simulink model "rlhighDynamicAcc"  (R2022b)
settings: Solver=ode4  StartTime=0.0  StopTime=inf  FixedStep=fixed_step_size  RelTol=1e-3  EnableMultiTasking=on
PreLoadFcn:
  | filepath  = fileparts(get_param(bdroot, 'FileName'))
  | cd(filepath);
InitFcn:
  | [filepath,name,ext] = fileparts(get_param(bdroot, 'FileName'));
  | InitFileName=[name,'_init.m'];
  | cd(filepath);
  | open_system(name);
  | % 命令旋钮
  | constant_block_path =[name '/cmd4UAVs'];
  | set_param(constant_block_path,'Value','0');
  | % 滑杆位置
  | constant_block_path = [name '/x_d'];
  | set_param(constant_block_path,'Value','0');
  | constant_block_path = [name '/y_d'];
  | set_param(constant_block_path,'Value','0');
  | constant_block_path = [name '/z_d'];
  | set_param(constant_block_path,'Value','-1.0');
  | constant_block_path = [name '/yaw_d'];
  | set_param(constant_block_path,'Value','0');
  | save_system(name);
  | try
  | run(InitFileName);
  | end
values from neighbouring files (symbols this model uses):
  MAX_ACC_HOR = 4.0    (= 4)    [rlhighDynamicAcc_init.m]
  MAX_POS_ERR = 4.0    (= 4)    [rlhighDynamicAcc_init.m]
  MAX_YAW_RATE = 1.0    (= 1)    [rlhighDynamicAcc_init.m]
  Pos_Y_I = 0.0    (= 0)    [rlhighDynamicAcc_init.m]
  Pos_Y_P = 1.0    (= 1)    [rlhighDynamicAcc_init.m]
  Pos_Z_P = 1.0    (= 1)    [rlhighDynamicAcc_init.m]
  Saturation_I_ah = 1.0    (= 1)    [rlhighDynamicAcc_init.m]
  Ts = fixed_step_size    (= 0.02)    [rlhighDynamicAcc_init.m]
  Vel_Y_I = 0.5    [rlhighDynamicAcc_init.m]
  Vel_Y_P = 2.0    (= 2)    [rlhighDynamicAcc_init.m]
  Yaw_I = 0.1    [rlhighDynamicAcc_init.m]
  Yaw_P = 1.0    (= 1)    [rlhighDynamicAcc_init.m]
undefined symbols (not defined in the file or in its folder): DiscIntNeverNeededParam
libraries: simulink x3, pixhawk_slib_swarm x3, rllib x1
settings Model: Creator=dream  LastModifiedBy=admin
settings SolverCC: AlgebraicLoopSolver=TrustRegion
settings DataIOCC: SaveFormat=Array  ReturnWorkspaceOutputs=off
settings OptimizationCC: BlockReduction=off  BooleanDataType=off  ZeroExternalMemoryAtStartup=off  ZeroInternalMemoryAtStartup=off
settings DebuggingCC: SaveWithParameterizedLinksMsg=none  UnderspecifiedInitializationDetection=Classic  MergeDetectMultiDrivingBlocksExec=none  SignalResolutionControl=TryResolveAllWithWarning  MultiTaskDSMMsg=warning  MultiTaskCondExecSysMsg=none  UnconnectedInputMsg=warning  UnconnectedOutputMsg=warning  UnconnectedLineMsg=warning  SFMachineParentedDataDiag=warning  ArithmeticOperatorsInVariantConditions=warning
settings HardwareCC: TargetBitPerPointer=64  TargetBitPerSizeT=64  TargetBitPerPtrDiffT=64  TargetLongLongMode=on  TargetIntDivRoundTo=Zero  TargetEndianess=LittleEndian  TargetWordSize=64  TargetHWDeviceType=MATLAB Host  ProdEqTarget=off
settings ModelReferenceCC: EnableRefExpFcnMdlSchedulingChecks=on  PropagateSignalLabelsOutOfModel=off
settings SFSimCC: SimUseLocalCustomCode=off  CustomCodeUndefinedFunction=UseInterfaceOnly  SimTargetLang=C++
settings RTWCC: PackageGeneratedCodeAndArtifacts=on  PackageName=RflyUdpExe  RTWUseLocalCustomCode=off  CustomLibrary=quat_mt.lib vrpn_mt.lib  BuildConfiguration=Faster Runs  TargetLang=C++
settings GRTTargetCC: TargetLangStandard=C++03 (ISO)  CodeInterfacePackaging=C++ class  MultiInstanceErrorCode=None

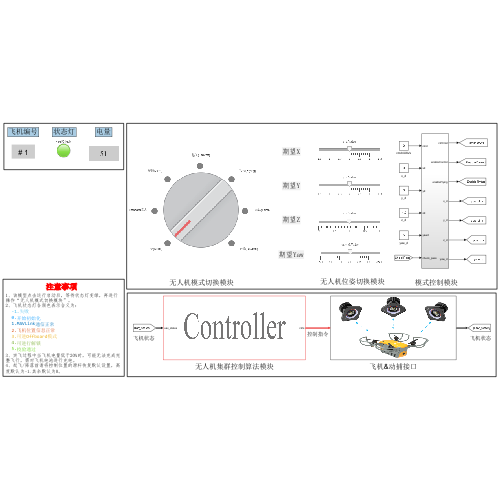
[thumbnail: Simulink's stored preview of the top-level diagram]
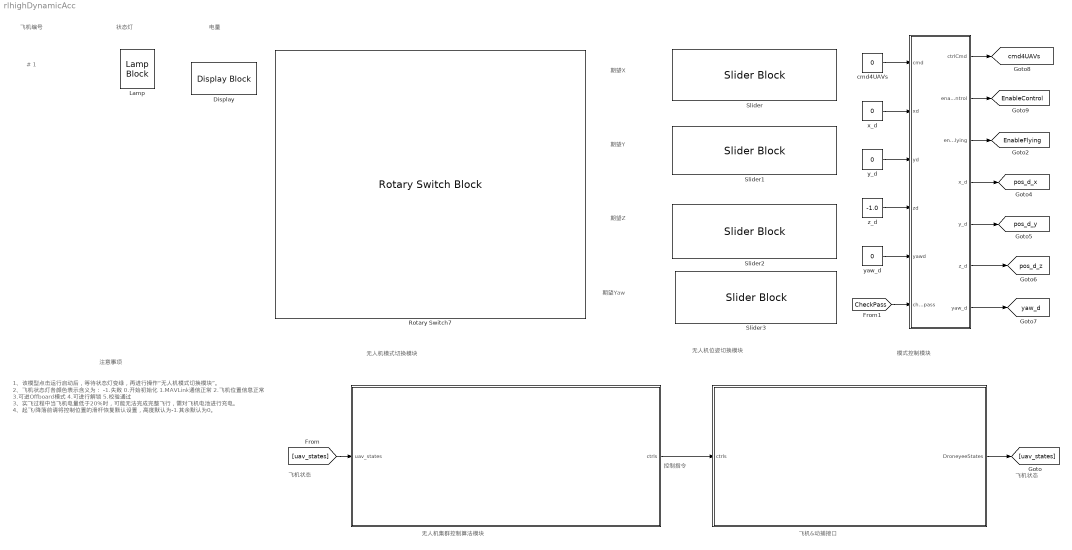
== system rlhighDynamicAcc ==
  note: 1、该模型点击运行启动后，等待状态灯变绿，再进行操作“无人机模式切换模块”。
      | 2、飞机状态灯各颜色表示含义为：
      | -1.失败
      | 0.开始初始化
      | 1.MAVLink通信正常
      | 2.飞机位置信息正常
      | 3.可进Offboard模式
      | 4.可进行解锁
      | 5.校验通过
      | 3、实飞过程中当飞机电量低于20%时，可能无法完成完整飞行，需对飞机电池进行充电。
      | 4、起飞/降落前请将控制位置的滑杆恢复默认设置，高度默认为-1.其余默认为0。
  note: 注意事项
  note: 控制指令
  note: 飞机&动捕接口
  note: 飞机编号
  note: 状态灯
  note: 电量
  note: # 1
  note: 无人机集群控制算法模块
  note: 飞机状态
  note: 模式控制模块
  note: 无人机模式切换模块
  note: 飞机状态
  note: 无人机位姿切换模块
  note: 期望Y
  note: 期望Z
  note: 期望X
  note: 期望Yaw
  " " : Subsystem
      mask Display: image('Controller.png');
  "   " : Subsystem
      mask Display: image('Odc_Sys.png');
  "    " : Subsystem
  Display : DisplayBlock  LabelPosition=Hide  Format=long
  Lamp : LampBlock
  Rotary Switch7 : RotarySwitchBlock  LabelPosition=Hide
      settings: Values={{'无(None)', 'Offboard模式', '解锁(Arm)', '起飞(Takeoff)', '飞行(Flying)', '着陆(Land)', '上锁(Disarm)'}, [0 8 4 256 512 1024 128]}
  Slider : SliderBlock  ScaleMin=-1.5  ScaleMax=1.5  TickInterval=0.5
  Slider1 : SliderBlock  ScaleMin=-1.5  ScaleMax=1.5  TickInterval=0.5
  Slider2 : SliderBlock  ScaleMin=-2  ScaleMax=0  TickInterval=0.5
  Slider3 : SliderBlock  ScaleMin=-3.1  ScaleMax=3.1  TickInterval=1
  cmd4UAVs : Constant  Value=0
  x_d : Constant  Value=0
  y_d : Constant  Value=0
  yaw_d : Constant  Value=0
  z_d : Constant  Value=-1.0
  tag scope: EnableControl=global, EnableFlying=global, cmd4UAVs=global, pos_d_x=global, pos_d_y=global, pos_d_z=global, yaw_d=global
  wires:
  " "/1(ctrls) -> "   "/1(ctrls)
  "   "/1(DroneyeeStates) -> [uav_states]
  [uav_states] -> " "/1(uav_states)
  "    "/6(z_d) -> [pos_d_z]
  "    "/3(enableFlying) -> [EnableFlying]
  "    "/2(enableControl) -> [EnableControl]
  "    "/1(ctrlCmd) -> [cmd4UAVs]
  [CheckPass] -> "    "/6(check_pass)
  "    "/4(x_d) -> [pos_d_x]
  z_d/1 -> "    "/4(zd)
  yaw_d/1 -> "    "/5(yawd)
  cmd4UAVs/1 -> "    "/1(cmd)
  y_d/1 -> "    "/3(yd)
  "    "/7(yaw_d) -> [yaw_d]
  "    "/5(y_d) -> [pos_d_y]
  x_d/1 -> "    "/2(xd)

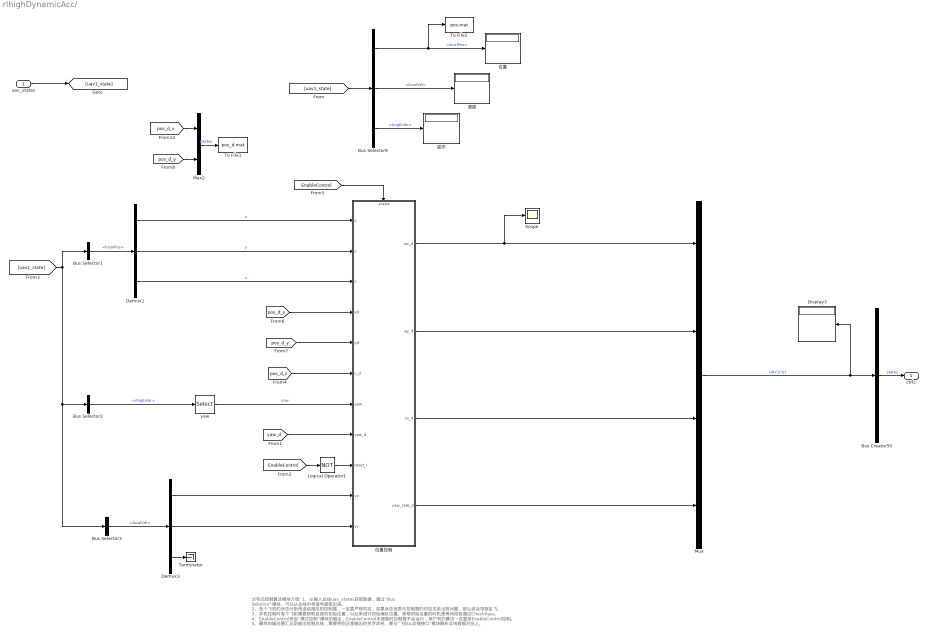
== system rlhighDynamicAcc/  ==
  note: 分布式控制算法模块介绍:
      |
      | 1、从输入总线uav_states获取数据，通过“Bus Selector”模块，可以从总线中将信号提取出来。
      | 2、各个飞机的状态分别传送给相应的控制器，一定要严格对应，如果状态信息与控制器的对应关系出现问题，那么就会导致乱飞。
      | 3、多机控制时每个飞机需要获取自身的初始位置，以此来进行初始编队位置。获取初始位置的时机是等待校验通过CheckPass。
      | 4、EnableControl来自“模式控制”模块的输出，EnableControl未使能时控制器不会运行，用户写的算法一定要受EnableControl控制。
      | 5、最终的输出要汇总到输出控制总线，需要特别注意输出的名字命名，要与“飞机&动捕接口”模块解析总线数据对应上。
  uav_states : Inport
  Bus Creator50 : BusCreator  Inputs=1
  Bus Selector1 : BusSelector  OutputSignals=localPos
  Bus Selector2 : BusSelector  OutputSignals=AngEular
  Bus Selector3 : BusSelector  OutputSignals=localVel
  Bus Selector9 : BusSelector  OutputSignals=localPos,localVel,AngEular
  Demux1 : Demux  Outputs=3
  Demux3 : Demux  Outputs=3
  Display3 : Display
  Logical Operator1 : Logic  Operator=NOT  AllPortsSameDT=off  OutDataTypeStr=boolean
  Mux : Mux
  Mux2 : Mux  Inputs=2
  Scope : Scope
  Terminator : Terminator
  To File1 : ToFile  Filename=pos_d.mat  SaveFormat=Timeseries
  To File2 : ToFile  Filename=pos.mat  SaveFormat=Timeseries
  yaw : Selector  InputPortWidth=3  IndexOptions=Index vector (dialog)  Indices=[3]  OutputSizes=1
  位置 : Display
  位置控制 : Subsystem
  姿态 : Display
  速度 : Display
  ctrls : Outport  VectorParamsAs1DForOutWhenUnconnected=off
  wires:
  Bus Creator50/1 -> ctrls/1  "states"
  Mux/1 -> Display3/1, Bus Creator50/1  "UAV1Ctrl"
  [uav1_state] -> Bus Selector1/1, Bus Selector3/1, Bus Selector2/1
  Demux1/1 -> 位置控制/1(x)  "x"
  Demux1/2 -> 位置控制/2(y)  "y"
  Demux1/3 -> 位置控制/3(z)  "z"
  Bus Selector1/1 -> Demux1/1  "<localPos>"
  yaw/1 -> 位置控制/7(yaw)  "yaw"
  Bus Selector2/1 -> yaw/1  "<AngEular>"
  位置控制/3(vz_d) -> Mux/3
  位置控制/4(yaw_rate_d) -> Mux/4
  Bus Selector9/3 -> 姿态/1  "<AngEular>"
  Bus Selector9/2 -> 速度/1  "<localVel>"
  Bus Selector9/1 -> To File2/1, 位置/1  "<localPos>"
  [uav1_state] -> Bus Selector9/1
  uav_states/1 -> [uav1_state]
  [EnableControl] -> 位置控制/Enable
  [yaw_d] -> 位置控制/8(yaw_d)
  [pos_d_z] -> 位置控制/6(z_d)
  [pos_d_y] -> 位置控制/5(yd)
  [pos_d_x] -> 位置控制/4(xd)
  Logical Operator1/1 -> 位置控制/9(reset_i)
  [EnableControl] -> Logical Operator1/1
  Demux3/3 -> Terminator/1
  Bus Selector3/1 -> Demux3/1  "<localVel>"
  Demux3/1 -> 位置控制/10(vx)
  Demux3/2 -> 位置控制/11(vy)
  位置控制/1(ax_d) -> Mux/1, Scope/1
  位置控制/2(ay_d) -> Mux/2
  [pos_d_x] -> Mux2/1
  [pos_d_y] -> Mux2/2
  Mux2/1 -> To File1/1  "states"

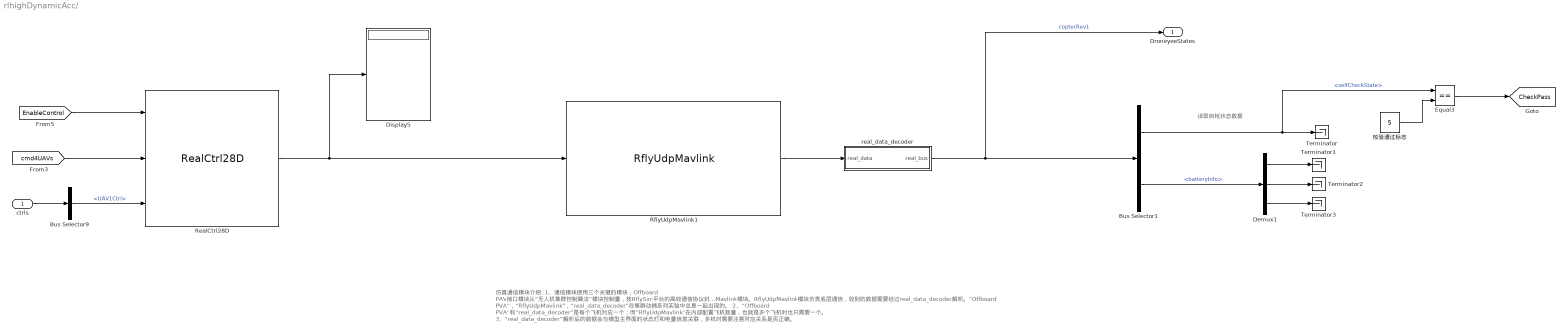
== system rlhighDynamicAcc/    ==
  note: 读取自检状态数据
  note: 仿真通信模块介绍:
      |
      | 1、通信模块使用三个关键的模块，Offboard PAV接口模块从“无人机集群控制算法”模块控制量，按RflySim平台的高效通信协议封装后传递给RflyUdpMavlink模块。RflyUdpMavlink模块负责底层通信，收到的数据需要经过real_data_decoder解析。“Offboard PVA”，“RflyUdpMavlink”，“real_data_decoder”在集群动捕系列实验中总是一起出现的。
      | 2、“Offboard PVA”和“real_data_decoder”是每个飞机对应一个；而“RflyUdpMavlink”在内部配置飞机数量，也就是多个飞机时也只需要一个。
      | 3、“real_data_decoder”解析后的数据会与模型主界面的状态灯和电量信息关联，多机时需要注意对应关系是否正确。
  ctrls : Inport
  Bus Selector1 : BusSelector  OutputSignals=selfCheckState,batteryInfo
  Bus Selector9 : BusSelector  OutputSignals=UAV1Ctrl
  Demux1 : Demux  Outputs=3
  Display5 : Display
  Equal3 : RelationalOperator  Operator===  OutDataTypeStr=boolean  RndMeth=Simplest  InputSameDT=off
  RealCtrl28D : pixhawk_slib_swarm/RealCtrl28D  isX=off  isY=off  isZ=off  isVx=off  isVy=off  isVz=on  isAx=on  isAy=on  isAz=off  isYaw=off  isYawRate=on  EnIdxList=[1]  isRcc=off  isForce=off  SamTime=-1
      settings: SourceProductName=Pixhawk Target Blocks
  RflyUdpMavlink1 : pixhawk_slib_swarm/RflyUdpMavlink  idx=1  ip1=127.0.0.1  ip=192.168.151.103  num=1  port=15501  Gps=[40.1540302,116.2593683,50.0]  udpmode=Mavlink_Real  T=1/50  isSame=off
      settings: SourceProductName=Pixhawk Target Blocks
  Terminator{,1..3} (4 alike) : Terminator
  real_data_decoder : Subsystem
      mask DialogControl Control2 Prompt: (Add text here)
  校验通过标志 : Constant  Value=5
  DroneyeeStates : Outport  VectorParamsAs1DForOutWhenUnconnected=off
  tag scope: CheckPass=global
  wires:
  RealCtrl28D/1 -> RflyUdpMavlink1/1, Display5/1
  RflyUdpMavlink1/1 -> real_data_decoder/1(real_data)
  real_data_decoder/1(real_bus) -> DroneyeeStates/1, Bus Selector1/1  "copterRev1"
  Bus Selector1/1 -> Equal3/1, Terminator/1  "<selfCheckState>"
  Demux1/3 -> Terminator3/1
  Demux1/2 -> Terminator2/1
  Demux1/1 -> Terminator1/1
  Bus Selector1/2 -> Demux1/1  "<batteryInfo>"
  Bus Selector9/1 -> RealCtrl28D/3  "<UAV1Ctrl>"
  [EnableControl] -> RealCtrl28D/1
  [cmd4UAVs] -> RealCtrl28D/2
  ctrls/1 -> Bus Selector9/1
  校验通过标志/1 -> Equal3/2
  Equal3/1 -> [CheckPass]

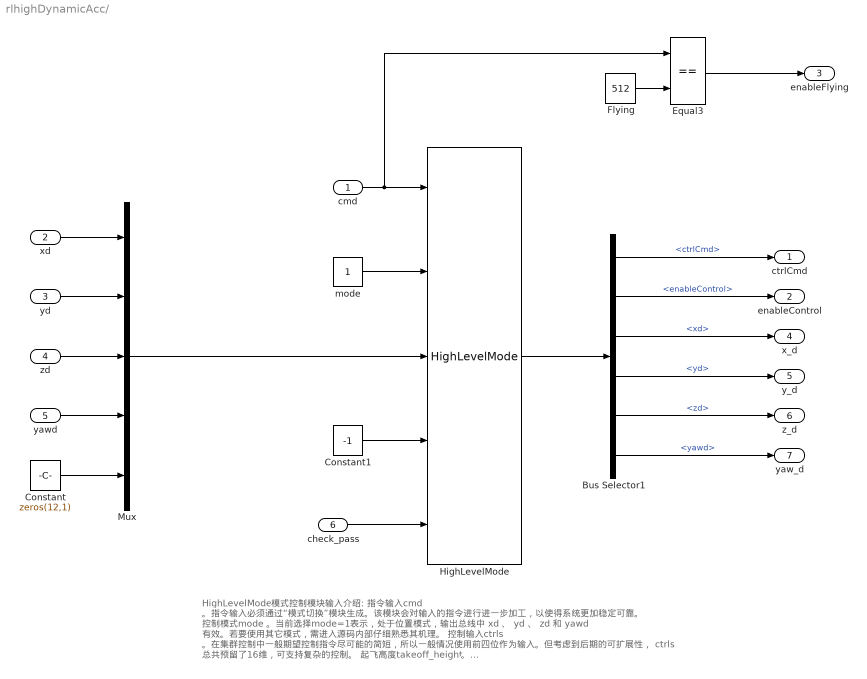
== system rlhighDynamicAcc/     ==
  note: HighLevelMode模式控制模块输入介绍:
      | 指令输入cmd 。指令输入必须通过“模式切换”模块生成。该模块会对输入的指令进行进一步加工，以使得系统更加稳定可靠。
      | 控制模式mode 。当前选择mode=1表示，处于位置模式，输出总线中 xd 、 yd 、 zd 和 yawd 有效。若要使用其它模式，需进入源码内部仔细熟悉其机理。
      | 控制输入ctrls 。在集群控制中一般期望控制指令尽可能的简短，所以一般情况使用前四位作为输入。但考虑到后期的可扩展性， ctrls 总共预留了16维，可支持复杂的控制。
      | 起飞高度takeoff_height。 起飞高度是指当用户将“模式切换”模块旋转到起飞时，飞机将自动起飞到的高度。该高度以向下为正，与无人机的 NED 坐标系兼容。在室内场景下，建议默认高度为1m，即在 MATLAB 中设置数值为-1。
      | 飞机状态校验是否通过check_pass 。 所有飞机校验通过才算通过，该信号来自飞机&动捕接口。
      | HighLevelMode模式控制模块输出介绍:
      | “模式控制”模块的输出是一个总线，MATLAB在从总线中提取数据时会显示总线中有哪些类型的数据，这样可以便于用户选择所需要的数据。
  cmd : Inport
  xd : Inport  Port=2
  yd : Inport  Port=3
  zd : Inport  Port=4
  yawd : Inport  Port=5
  check_pass : Inport  Port=6
  Bus Selector1 : BusSelector  OutputSignals=ctrlCmd,enableControl,xd,yd,zd,yawd
  Constant : Constant  Value=zeros(12,1)
  Constant1 : Constant  Value=-1
  Equal3 : RelationalOperator  Operator===  OutDataTypeStr=boolean  RndMeth=Simplest  InputSameDT=off
  Flying : Constant  Value=512
  HighLevelMode : pixhawk_slib_swarm/HighLevelMode
      settings: SourceProductName=Pixhawk Target Blocks
  Mux : Mux  Inputs=5
  mode : Constant
  ctrlCmd : Outport  VectorParamsAs1DForOutWhenUnconnected=off
  enableControl : Outport  Port=2  VectorParamsAs1DForOutWhenUnconnected=off
  enableFlying : Outport  Port=3  VectorParamsAs1DForOutWhenUnconnected=off
  x_d : Outport  Port=4  VectorParamsAs1DForOutWhenUnconnected=off
  y_d : Outport  Port=5  VectorParamsAs1DForOutWhenUnconnected=off
  z_d : Outport  Port=6  VectorParamsAs1DForOutWhenUnconnected=off
  yaw_d : Outport  Port=7  VectorParamsAs1DForOutWhenUnconnected=off
  wires:
  Mux/1 -> HighLevelMode/3
  Bus Selector1/5 -> z_d/1  "<zd>"
  Bus Selector1/3 -> x_d/1  "<xd>"
  Bus Selector1/2 -> enableControl/1  "<enableControl>"
  Constant1/1 -> HighLevelMode/4
  Bus Selector1/1 -> ctrlCmd/1  "<ctrlCmd>"
  yawd/1 -> Mux/4
  HighLevelMode/1 -> Bus Selector1/1
  Constant/1 -> Mux/5
  check_pass/1 -> HighLevelMode/5
  xd/1 -> Mux/1
  zd/1 -> Mux/3
  Bus Selector1/4 -> y_d/1  "<yd>"
  mode/1 -> HighLevelMode/2
  yd/1 -> Mux/2
  Bus Selector1/6 -> yaw_d/1  "<yawd>"
  Equal3/1 -> enableFlying/1
  Flying/1 -> Equal3/2
  cmd/1 -> Equal3/1, HighLevelMode/1

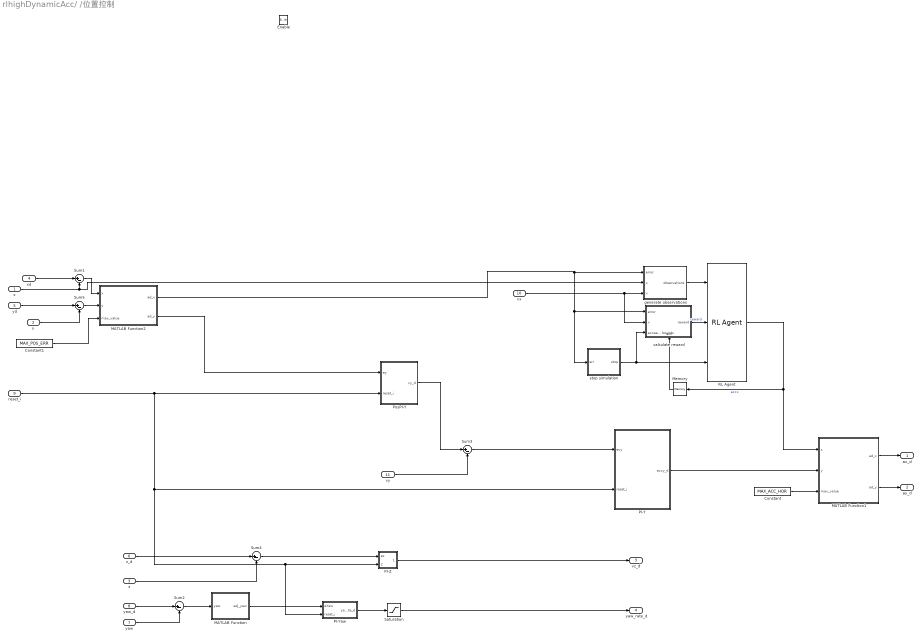
== system rlhighDynamicAcc/ /位置控制 ==
  x : Inport
  y : Inport  Port=2
  z : Inport  Port=3
  xd : Inport  Port=4
  yd : Inport  Port=5
  z_d : Inport  Port=6
  yaw : Inport  Port=7
  yaw_d : Inport  Port=8
  reset_i : Inport  Port=9
  vx : Inport  Port=10
  vy : Inport  Port=11
  Enable : EnablePort
  Constant : Constant  Value=MAX_ACC_HOR
  Constant1 : Constant  Value=MAX_POS_ERR
  MATLAB Function : MATLAB Function  TreatAsAtomicUnit=on
  MATLAB Function1 : MATLAB Function  TreatAsAtomicUnit=on
  MATLAB Function2 : MATLAB Function  TreatAsAtomicUnit=on
  Memory : Memory
  PI-Y : Subsystem
  PI-Yaw : Subsystem
  PI-Z : Subsystem
  PosPI-Y : Subsystem
  RL Agent : rllib/RL Agent  Agent=agent  ExternalActionAsInput=off  ProvideLastAction=off  ProvideCumRwd=off  TreatAsDirectFeedthrough=on  UseStrictObservationDataTypes=off
  Saturation : Saturate  UpperLimit=MAX_YAW_RATE  LowerLimit=-MAX_YAW_RATE
  Sum{1..5} (5 alike) : Sum  Inputs=|+-
  calculate reward : Subsystem
      settings: PortSchema="{\"entries\":[{\"content\":{\"sides\":[{\"content\":{\"connectorIds\":[\"In1\",\"In2\",\"In3\"]},\"type\":\"ConnectorPlacement.EquallySpacedRectSide\",\"uuid\":\"a6831b4c-c5e4-4b81-8e40-7fc4b7dad633\"},{\"content\":{\"connectorIds\":[\"Out1\"],\"side\":\"RIGHT\"},\"type\":\"ConnectorPlacement.EquallySpacedRectSide\",\"uuid\":\"8e922aec-ef45-4070-9445-bf1f36bf8a17\"},{\"content\":{\"connectorIds\":[],\"side\":\"TOP\"},\"type\":\"ConnectorPlacement.EquallySpacedRectSide\",\"uuid\":\"70fa4f95-2353-478a-a00d-3d58ec9167ce\"},{\"content\":{\"connectorIds\":[\"In4\"],\"side\":\"BOTTOM\"},\"type\":\"ConnectorPlacement.EquallySpacedRectSide\",\"uuid\":\"92073c7e-e113-4538-8fec-17539d6aadbe\"}]},\"type\":\"ConnectorPlacement.EquallySpacedConnector\",\"uuid\":\"a5a5b4e0-4f16-4179-a493-15187e3b2ccc\"}],\"packageUris\":[\"http://schema.mathworks.com/mf0/Connector/R2020b\"],\"version\":\"1.0\"}"
  generate observations : Subsystem
  stop simulation : Subsystem
  ax_d : Outport  VectorParamsAs1DForOutWhenUnconnected=off
  ay_d : Outport  Port=2  VectorParamsAs1DForOutWhenUnconnected=off
  vz_d : Outport  Port=3  VectorParamsAs1DForOutWhenUnconnected=off
  yaw_rate_d : Outport  Port=4  VectorParamsAs1DForOutWhenUnconnected=off
  wires:
  yaw_d/1 -> Sum2/1
  MATLAB Function/1(adj_yaw) -> PI-Yaw/1(eYaw)
  PI-Yaw/1(yawRate_d) -> Saturation/1
  z_d/1 -> Sum4/1
  PI-Z/1(vy_d) -> vz_d/1
  Saturation/1 -> yaw_rate_d/1
  z/1 -> Sum4/2
  yaw/1 -> Sum2/2
  Sum4/1 -> PI-Z/1(ez)
  Sum2/1 -> MATLAB Function/1(yaw)
  MATLAB Function1/1(ad_x) -> ax_d/1
  MATLAB Function1/2(ad_y) -> ay_d/1
  vy/1 -> Sum3/2
  Sum3/1 -> PI-Y/1(evy)
  PosPI-Y/1(vy_d) -> Sum3/1
  PI-Y/1(accy_d) -> MATLAB Function1/2(y)
  Constant/1 -> MATLAB Function1/3(max_value)
  Constant1/1 -> MATLAB Function2/3(max_value)
  xd/1 -> Sum1/1
  yd/1 -> Sum5/1
  Sum5/1 -> MATLAB Function2/2(y)
  Sum1/1 -> MATLAB Function2/1(x)
  MATLAB Function2/2(ad_y) -> PosPI-Y/1(ey)
  x/1 -> generate observations/2(x), Sum1/2
  reset_i/1 -> PI-Z/2(reset_i), PI-Yaw/2(reset_i), PI-Y/2(reset_i), PosPI-Y/2(reset_i)
  y/1 -> Sum5/2
  vx/1 -> calculate reward/2(v), generate observations/3(v)
  MATLAB Function2/1(ad_x) -> generate observations/1(error), calculate reward/1(error), stop simulation/1(err)
  generate observations/1(observations) -> RL Agent/1
  stop simulation/1(stop) -> calculate reward/3(exceeds bounds), RL Agent/3
  RL Agent/1 -> MATLAB Function1/1(x), Memory/1  "accx"
  calculate reward/1(reward) -> RL Agent/2  "reward"
  Memory/1 -> calculate reward/4(acc)

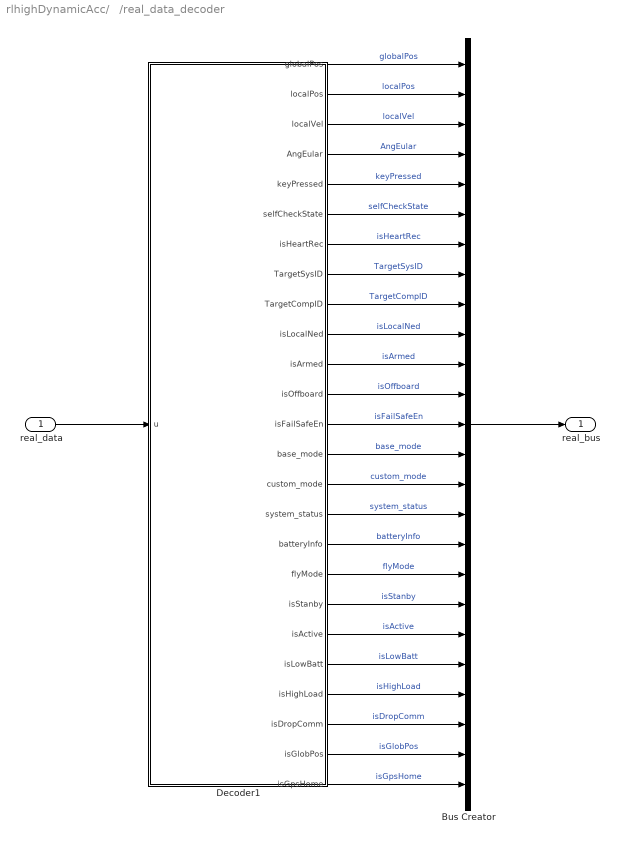
== system rlhighDynamicAcc/   /real_data_decoder ==
  real_data : Inport
  Bus Creator : BusCreator  Inputs=25
  Decoder1 : MATLAB Function  TreatAsAtomicUnit=on
  real_bus : Outport  VectorParamsAs1DForOutWhenUnconnected=off
  wires:
  Decoder1/3(localVel) -> Bus Creator/3  "localVel"
  Decoder1/15(custom_mode) -> Bus Creator/15  "custom_mode"
  Decoder1/21(isLowBatt) -> Bus Creator/21  "isLowBatt"
  Decoder1/9(TargetCompID) -> Bus Creator/9  "TargetCompID"
  Decoder1/18(flyMode) -> Bus Creator/18  "flyMode"
  Decoder1/16(system_status) -> Bus Creator/16  "system_status"
  Decoder1/5(keyPressed) -> Bus Creator/5  "keyPressed"
  real_data/1 -> Decoder1/1(u)
  Bus Creator/1 -> real_bus/1
  Decoder1/14(base_mode) -> Bus Creator/14  "base_mode"
  Decoder1/22(isHighLoad) -> Bus Creator/22  "isHighLoad"
  Decoder1/25(isGpsHome) -> Bus Creator/25  "isGpsHome"
  Decoder1/24(isGlobPos) -> Bus Creator/24  "isGlobPos"
  Decoder1/19(isStanby) -> Bus Creator/19  "isStanby"
  Decoder1/20(isActive) -> Bus Creator/20  "isActive"
  Decoder1/12(isOffboard) -> Bus Creator/12  "isOffboard"
  Decoder1/10(isLocalNed) -> Bus Creator/10  "isLocalNed"
  Decoder1/8(TargetSysID) -> Bus Creator/8  "TargetSysID"
  Decoder1/13(isFailSafeEn) -> Bus Creator/13  "isFailSafeEn"
  Decoder1/4(AngEular) -> Bus Creator/4  "AngEular"
  Decoder1/11(isArmed) -> Bus Creator/11  "isArmed"
  Decoder1/23(isDropComm) -> Bus Creator/23  "isDropComm"
  Decoder1/7(isHeartRec) -> Bus Creator/7  "isHeartRec"
  Decoder1/17(batteryInfo) -> Bus Creator/17  "batteryInfo"
  Decoder1/6(selfCheckState) -> Bus Creator/6  "selfCheckState"
  Decoder1/1(globalPos) -> Bus Creator/1  "globalPos"
  Decoder1/2(localPos) -> Bus Creator/2  "localPos"

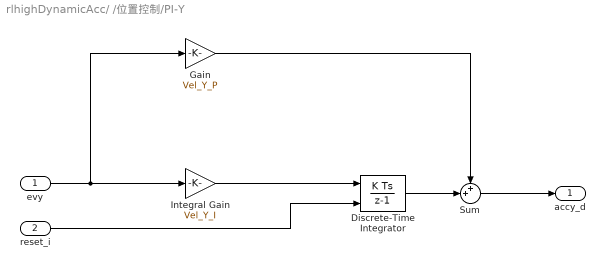
== system rlhighDynamicAcc/ /位置控制/PI-Y ==
  evy : Inport
  reset_i : Inport  Port=2
  Discrete-Time Integrator : DiscreteIntegrator  ExternalReset=level  SampleTime=-1  LimitOutput=on  UpperSaturationLimit=Saturation_I_ah  LowerSaturationLimit=-Saturation_I_ah  ICPrevOutput=DiscIntNeverNeededParam  ICPrevScaledInput=DiscIntNeverNeededParam
  Gain : Gain  Gain=Vel_Y_P
  Integral Gain : Gain  DisableCoverage=on  Gain=Vel_Y_I
  Sum : Sum  Inputs=++|
  accy_d : Outport  InitialOutput=0  VectorParamsAs1DForOutWhenUnconnected=off
  wires:
  evy/1 -> Gain/1, Integral Gain/1
  Integral Gain/1 -> Discrete-Time Integrator/1
  Gain/1 -> Sum/1
  Sum/1 -> accy_d/1
  Discrete-Time Integrator/1 -> Sum/2
  reset_i/1 -> Discrete-Time Integrator/2

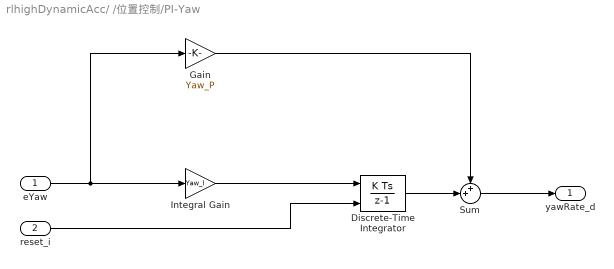
== system rlhighDynamicAcc/ /位置控制/PI-Yaw ==
  eYaw : Inport
  reset_i : Inport  Port=2
  Discrete-Time Integrator : DiscreteIntegrator  ExternalReset=level  SampleTime=-1  LimitOutput=on  UpperSaturationLimit=Saturation_I_ah  LowerSaturationLimit=-Saturation_I_ah  ICPrevOutput=DiscIntNeverNeededParam  ICPrevScaledInput=DiscIntNeverNeededParam
  Gain : Gain  Gain=Yaw_P
  Integral Gain : Gain  DisableCoverage=on  Gain=Yaw_I
  Sum : Sum  Inputs=++|
  yawRate_d : Outport  InitialOutput=0  VectorParamsAs1DForOutWhenUnconnected=off
  wires:
  eYaw/1 -> Gain/1, Integral Gain/1
  Integral Gain/1 -> Discrete-Time Integrator/1
  Gain/1 -> Sum/1
  Sum/1 -> yawRate_d/1
  Discrete-Time Integrator/1 -> Sum/2
  reset_i/1 -> Discrete-Time Integrator/2

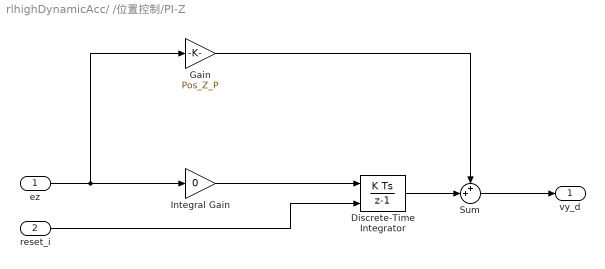
== system rlhighDynamicAcc/ /位置控制/PI-Z ==
  ez : Inport
  reset_i : Inport  Port=2
  Discrete-Time Integrator : DiscreteIntegrator  ExternalReset=level  SampleTime=-1  LimitOutput=on  UpperSaturationLimit=Saturation_I_ah  LowerSaturationLimit=-Saturation_I_ah  ICPrevOutput=DiscIntNeverNeededParam  ICPrevScaledInput=DiscIntNeverNeededParam
  Gain : Gain  Gain=Pos_Z_P
  Integral Gain : Gain  DisableCoverage=on  Gain=0
  Sum : Sum  Inputs=++|
  vy_d : Outport  InitialOutput=0  VectorParamsAs1DForOutWhenUnconnected=off
  wires:
  ez/1 -> Gain/1, Integral Gain/1
  Integral Gain/1 -> Discrete-Time Integrator/1
  Gain/1 -> Sum/1
  Sum/1 -> vy_d/1
  Discrete-Time Integrator/1 -> Sum/2
  reset_i/1 -> Discrete-Time Integrator/2

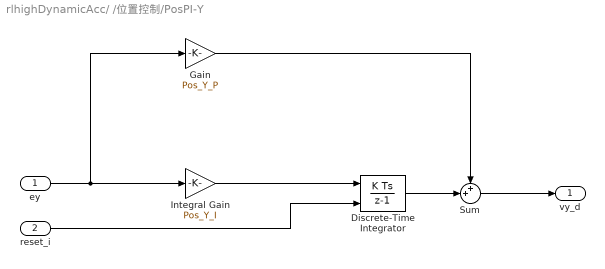
== system rlhighDynamicAcc/ /位置控制/PosPI-Y ==
  ey : Inport
  reset_i : Inport  Port=2
  Discrete-Time Integrator : DiscreteIntegrator  ExternalReset=level  SampleTime=-1  LimitOutput=on  UpperSaturationLimit=Saturation_I_ah  LowerSaturationLimit=-Saturation_I_ah  ICPrevOutput=DiscIntNeverNeededParam  ICPrevScaledInput=DiscIntNeverNeededParam
  Gain : Gain  Gain=Pos_Y_P
  Integral Gain : Gain  DisableCoverage=on  Gain=Pos_Y_I
  Sum : Sum  Inputs=++|
  vy_d : Outport  InitialOutput=0  VectorParamsAs1DForOutWhenUnconnected=off
  wires:
  ey/1 -> Gain/1, Integral Gain/1
  Integral Gain/1 -> Discrete-Time Integrator/1
  Gain/1 -> Sum/1
  Sum/1 -> vy_d/1
  Discrete-Time Integrator/1 -> Sum/2
  reset_i/1 -> Discrete-Time Integrator/2

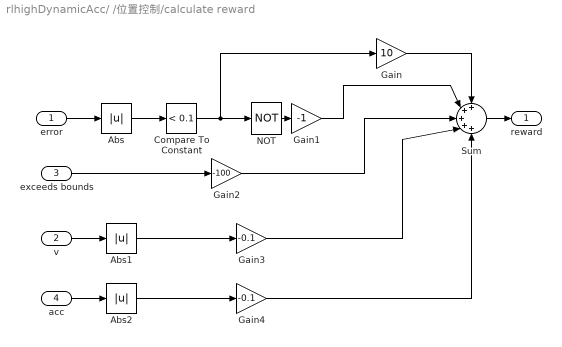
== system rlhighDynamicAcc/ /位置控制/calculate reward ==
  error : Inport
  v : Inport  Port=2
  exceeds bounds : Inport  Port=3
  acc : Inport  Port=4
  Abs : Abs  SaturateOnIntegerOverflow=off
  Abs1 : Abs  ZeroCross=off  SaturateOnIntegerOverflow=off
  Abs2 : Abs  ZeroCross=off  SaturateOnIntegerOverflow=off
  Compare To Constant : simulink/Logic and Bit Operations/Compare To Constant  relop=<  const=0.1  OutDataTypeStr=boolean
  Gain : Gain  Gain=10
  Gain1 : Gain  Gain=-1
  Gain2 : Gain  Gain=-100
  Gain3 : Gain  Gain=-0.1
  Gain4 : Gain  Gain=-0.1
  NOT : Logic  Operator=NOT  IconShape=distinctive  AllPortsSameDT=off  OutDataTypeStr=boolean
  Sum : Sum  Inputs=+++++  OutDataTypeStr=double
  reward : Outport  VectorParamsAs1DForOutWhenUnconnected=off
  wires:
  Abs/1 -> Compare To Constant/1
  Gain2/1 -> Sum/3
  Gain/1 -> Sum/1
  Compare To Constant/1 -> NOT/1, Gain/1
  Gain1/1 -> Sum/2
  Sum/1 -> reward/1
  NOT/1 -> Gain1/1
  exceeds bounds/1 -> Gain2/1
  error/1 -> Abs/1
  v/1 -> Abs1/1
  Gain3/1 -> Sum/4
  Abs1/1 -> Gain3/1
  Abs2/1 -> Gain4/1
  acc/1 -> Abs2/1
  Gain4/1 -> Sum/5

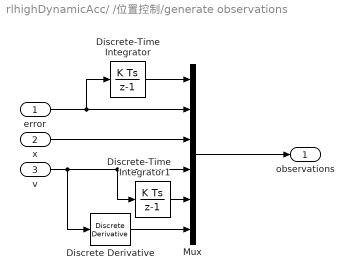
== system rlhighDynamicAcc/ /位置控制/generate observations ==
  error : Inport
  x : Inport  Port=2
  v : Inport  Port=3
  Discrete Derivative : simulink/Discrete/Discrete Derivative  gainval=0.01  ICPrevScaledInput=0.0  OutMin=[]  OutMax=[]  OutDataType=fixdt(1, 16)  OutScaling=2^-10  DoSatur=off
  Discrete-Time Integrator : DiscreteIntegrator  SampleTime=Ts  ICPrevOutput=DiscIntNeverNeededParam  ICPrevScaledInput=DiscIntNeverNeededParam
  Discrete-Time Integrator1 : DiscreteIntegrator  gainval=0.1  SampleTime=Ts  ICPrevOutput=DiscIntNeverNeededParam  ICPrevScaledInput=DiscIntNeverNeededParam
  Mux : Mux  Inputs=6
  observations : Outport  VectorParamsAs1DForOutWhenUnconnected=off
  wires:
  x/1 -> Mux/3
  Discrete-Time Integrator/1 -> Mux/1
  error/1 -> Discrete-Time Integrator/1, Mux/2
  Mux/1 -> observations/1
  v/1 -> Discrete Derivative/1, Discrete-Time Integrator1/1, Mux/4
  Discrete-Time Integrator1/1 -> Mux/5
  Discrete Derivative/1 -> Mux/6

== system rlhighDynamicAcc/ /位置控制/stop simulation ==
  err : Inport
  Abs : Abs  SaturateOnIntegerOverflow=off
  Compare To Constant : simulink/Logic and Bit Operations/Compare To Constant  relop=>  const=10  OutDataTypeStr=boolean
  stop : Outport  VectorParamsAs1DForOutWhenUnconnected=off
  wires:
  err/1 -> Abs/1
  Abs/1 -> Compare To Constant/1
  Compare To Constant/1 -> stop/1

== matlab function rlhighDynamicAcc/   /real_data_decoder/Decoder1 ==
  data: u input; globalPos output; localPos output; localVel output; AngEular output; keyPressed output; selfCheckState output; isHeartRec output; TargetSysID output; TargetCompID output; isLocalNed output; isArmed output; isOffboard output; isFailSafeEn output; base_mode output; custom_mode output; system_status output; batteryInfo output; flyMode output; isStanby output; isActive output; isLowBatt output; isHighLoad output; isDropComm output; isGlobPos output; isGpsHome output
function [globalPos,localPos,localVel,AngEular,keyPressed,selfCheckState,isHeartRec,TargetSysID,TargetCompID,isLocalNed,isArmed,isOffboard,isFailSafeEn,base_mode,custom_mode,system_status,batteryInfo,flyMode,isStanby,isActive,isLowBatt,isHighLoad,isDropComm,isGlobPos,isGpsHome] = fcn(u)

globalPos=u(1:3);  % CopterSim全局位置，单位m。根据飞机的GPS坐标解算得到，以Ue地图的坐标中心为原点，使用多机控制时，应该使用本接口。
AngEular=u(4:6); %Pixhawk估计得到的姿态欧拉角，单位弧度
localPos=u(7:9); %Pixhawk估计得到的以gpsHome为原点的相对北东地位置向量，单位m，z轴向下为正
localVel=u(10:12); %北东地的运动速度向量，单位m/s

keyPressed=u(13);
selfCheckState=u(14);
isHeartRec=u(15);
TargetSysID=u(16);
TargetCompID=u(17);
isLocalNed=u(18);
isArmed=u(19);
isOffboard=u(20);
isFailSafeEn=u(21);
base_mode=u(22);
custom_mode=u(23);
system_status=u(24);
batteryInfo=u(25:27); %3D

flyMode=u(28);
isStanby=u(29);
isActive=u(30);
isLowBatt=u(31);
isHighLoad=u(32);
isDropComm=u(33);
isGlobPos=u(34);
isGpsHome=u(35);

== matlab function rlhighDynamicAcc/ /位置控制/MATLAB Function ==
  data: yaw input; adj_yaw output
% 动捕偏航角与PX4偏航角的差值
function adj_yaw  = limit_yaw(yaw)
if abs(yaw)>pi
    if yaw>0
        adj_yaw=yaw-2*pi;
    else
        adj_yaw=2*pi+yaw;
    end
else
    adj_yaw=yaw;
end

== matlab function rlhighDynamicAcc/ /位置控制/MATLAB Function1 ==
  data: x input; ad_x output; y input; ad_y output; max_value input
% 限制水平幅度
function [ad_x, ad_y]  = limit(x, y, max_value)
a = sqrt(x*x+y*y);
ad_x = x;
ad_y = y;
if (a > max_value)
    ad_x = x/a*max_value;
    ad_y = y/a*max_value;
end

== matlab function rlhighDynamicAcc/ /位置控制/MATLAB Function2 ==
  data: x input; ad_x output; y input; ad_y output; max_value input
% 限制水平幅度
function [ad_x, ad_y]  = limit(x, y, max_value)
a = sqrt(x*x+y*y);
ad_x = x;
ad_y = y;
if (a > max_value)
    ad_x = x/a*max_value;
    ad_y = y/a*max_value;
end
